simulink library "inp"  (R2021b)
settings: Solver=VariableStepAuto  StartTime=0.0  StopTime=10.0  RelTol=1e-3
undefined symbols (not defined in the file): C_TASK_5MS_S, FALSE, KINP_AcoreReadyToSlp_flg_ovrdflg, KINP_AcoreReadyToSlp_flg_ovrdval, KINP_AllowMovThd_OTA_enum_ovrdflg, KINP_AllowMovThd_OTA_enum_ovrdval, KINP_APSAngleTarget_Deg_ovrdflg, KINP_APSAngleTarget_Deg_ovrdval, KINP_APSDecReq_mps2_ovrdflg, KINP_APSDecReq_mps2_ovrdval, KINP_APSDecReqA_flg_ovrdflg, KINP_APSDecReqA_flg_ovrdval, KINP_APSDFLL_cm_ovrdflg, KINP_APSDFLL_cm_ovrdval, KINP_APSDFLR_cm_ovrdflg, KINP_APSDFLR_cm_ovrdval, KINP_APSDRLL_cm_ovrdflg, KINP_APSDRLL_cm_ovrdval, KINP_APSDRLR_cm_ovrdflg, KINP_APSDRLR_cm_ovrdval, KINP_APSExitCondition_enum_ovrdflg, KINP_APSExitCondition_enum_ovrdval, KINP_APSHWVer_enum_ovrdflg, KINP_APSHWVer_enum_ovrdval, KINP_APSProgressPCT_pct_ovrdflg, KINP_APSProgressPCT_pct_ovrdval, KINP_APSPwrReq_enum_ovrdflg, KINP_APSPwrReq_enum_ovrdval, KINP_APSReq_enum_ovrdflg, KINP_APSReq_enum_ovrdval, KINP_APSRQDisplay_enum_ovrdflg, KINP_APSRQDisplay_enum_ovrdval, KINP_APSRqEPASCtrl_flg_ovrdflg, KINP_APSRqEPASCtrl_flg_ovrdval, KINP_APSShiftPosnReq_enum_ovrdval, KINP_APSShiftPosnReq_enum_ovrflg, KINP_APSSpeedCMD_kph_ovrdval, KINP_APSSpeedCMD_kph_ovrflg, KINP_APSStaSystem_enum_ovrdflg, KINP_APSStaSystem_enum_ovrdval, KINP_APSSWVer_enum_ovrdflg, KINP_APSSWVer_enum_ovrdval, KINP_APSVMCReqA_flg_ovrdval, KINP_APSVMCReqA_flg_ovrflg, KINP_APSVRqEPASCtrl_flg_ovrdflg, KINP_APSVRqEPASCtrl_flg_ovrdval, KINP_AuxBattVolmV_mV_ovrdflg, KINP_AuxBattVolmV_mV_ovrdval, KINP_BTConnectSta_enum_ovrdflg, KINP_BTConnectSta_enum_ovrdval, KINP_CAASSta_enum_ovrdflg, KINP_CAASSta_enum_ovrdval, KINP_CAASVMCReqA_flg_ovrdval, KINP_CAASVMCReqA_flg_ovrflg, KINP_CAN1BusOff_flg_ovrdflg, KINP_CAN1BusOff_flg_ovrdval, KINP_CAN2BusOff_flg_ovrdflg, KINP_CAN2BusOff_flg_ovrdval, KINP_CAN3BusOff_flg_ovrdflg, KINP_CAN3BusOff_flg_ovrdval ... (+222)
libraries: FVT_lib x1035, hcu_lib x1
(part 9 of 33)

== system inp/INP/CAN4/CreateBus ==
  inp_CanValid_bus : Inport
  inp_Hal_bus : Inport  Port=2
  UnitConverter_{1..21,28..30,35,38,45..46,63,65,70..71,74,79..81,83,85..86,88..91,114..116,118..119,121..138,140..142,157,189,192,196..198,201..202,205..206,209..210,213..214,216..250,259..261,267} (122 alike) : DataTypeConversion  OutDataTypeStr=boolean
  UnitConverter_{22..25,31..34,36..37,41..42,47..62,64,69,72..73,76..78,87,94,96,98,100,102,104,106,108,110,112..113,139,147,149,151..156,159,161,163,165,167,169,171,173..177,179,190..191,193..195,200,204,208,212,215,251..258,263,265..266,269,271..272} (93 alike) : DataTypeConversion  OutDataTypeStr=uint8
  UnitConverter_{26..27,40,43..44,75,82,84,93,95,97,99,101,103,105,107,109,111,117,120,143..146,148,150,158,160,162,164,166,168,170,172,178,180..188,199,203,207,211} (48 alike) : DataTypeConversion  OutDataTypeStr=single
  UnitConverter_{39,92,262,264,268,270} (6 alike) : DataTypeConversion  OutDataTypeStr=uint16
  UnitConverter_66 : DataTypeConversion  OutDataTypeStr=uint64
  UnitConverter_67 : DataTypeConversion  OutDataTypeStr=uint64
  UnitConverter_68 : DataTypeConversion  OutDataTypeStr=uint64
  bus_creator : BusCreator  Inputs=272  OutDataTypeStr=Bus: BINP_CAN4_outputs  NonVirtualBus=on
  bus_selector : BusSelector  OutputSignals=VINP_CANMsgValidBodyZoneDR1_flg,VINP_CANMsgValidBodyZoneDR2_flg,VINP_CANMsgValidBodyZonePS1_flg,VINP_CANMsgValidBodyZonePS2_flg,VINP_CANMsgValidDKC1_flg,VINP_CANMsgValidDKC2_flg,VINP_CANMsgValidPTG1_flg,VINP_CANMsgValidZONEDR1_flg,VINP_CANMsgValidZONEDRVCU_flg,VINP_CANMsgValidZONEFR1_flg,VINP_CANMsgValidZONEFRVCU_flg,VINP_CANMsgValidzGWAPTC1_flg,VINP_CANMsgValidzGWCANFr1_flg,VINP_CANMsgValidzGWLINDr1_flg,VINP_CANMsgValidzGWLINDr2_flg,VINP_CANMsgValidzGWLINFr1_flg,VINP_CANMsgValidzGWLINFr2_flg,VINP_CANMsgValidzGWSEAT1_flg
  bus_selector_1 : BusSelector  OutputSignals=VINP_BDDSEATAntiSta_flg,VINP_BDDSEATEntryFunSta_flg,VINP_BDDSEATErrorSta_flg,VINP_BDDSEATMemSetSta_enum,VINP_BDDSEATModeSta_enum,VINP_BDDSEATVentSta_enum,VINP_BDDSEATheaterSta_enum,VINP_BDAPMWinFOpenedSta_pct,VINP_BDAPMWinROpenedSta_pct,VINP_BDDoorFHandleCloseSta_flg,VINP_BDDoorRHandleCloseSta_flg,VINP_BPPSEATErrorSta_flg,VINP_BPPSEATModeSta_enum,VINP_BPPSEATVentSta_enum,VINP_BPPSEATheaterSta_enum,VINP_BPPTGActiveSta_enum,VINP_BPPTGExistSta_flg,VINP_BPPTGInsideSW1Sta_enum,VINP_BPPTGInsideSW2Sta_enum,VINP_BPPTGIsSetHeightSta_flg,VINP_BPPTGLeftHallPosnSta_enum,VINP_BPPTGOpenRatioSta_pct,VINP_BPPTGRDILCmd_enum,VINP_BPPTGSysSta_enum,VINP_BPAPMWinFOpenedSta_pct,VINP_BPAPMWinROpenedSta_pct,VINP_BPDoorFHandleCloseSta_flg,VINP_BPDoorRHandleCloseSta_flg,VINP_BPSEATLVentSta_enum,VINP_BPSEATMLVentSta_enum,VINP_BPSEATMRVentSta_enum,VINP_BPSEATRVentSta_enum,VINP_DKCKeyNumSta_enum,VINP_DKCKeyTypeSta_enum,VINP_DKCPDkeyAreaRAPSSta_enum,VINP_DKCParkingModeCmd_enum,VINP_DKCReVehData_enum,VINP_PCommandToBCM_enum,VINP_PCommandToPTG_enum,VINP_PDKeyAreaLockUnlock_enum,VINP_PDKeyAreaPS_enum,VINP_PDKeyAreaPTG_enum,VINP_PDKeyWelcome_enum,VINP_PDkeyShowIVI_enum,VINP_PKeyMiss_flg,VINP_PKeyMode_enum,VINP_PUIDLowPower_flg,VINP_EncryptionDATA063_enum,VINP_EncryptionDATA64127_enum,VINP_RandomNumberX_enum,VINP_PTGActiveSta_enum,VINP_PTGAutoStaus_flg,VINP_PTGExist_flg,VINP_PTGHWVer_enum,VINP_PTGInnerSW2_enum,VINP_PTGIsSetHeight_flg,VINP_PTGOpenRatio_pct,VINP_PTGRDILSta_enum,VINP_PTGSWVer_enum,VINP_PTGSysSta_enum,VINP_DrLockSta_flg,VINP_MIRRORFOLDSW_flg,VINP_RLTurnLPErr_flg,VINP_RLTurnLampC_mA,VINP_RRTurnLPErr_flg,VINP_RRTurnLampC_mA,VINP_RWiperAS_flg,VINP_RWiperProtection_flg,VINP_BlowerErr_enum,VINP_DrPMMLVOutPErrLmp_flg,VINP_DrPMMSysErrLmp_flg,VINP_DrSCPSysErrLmp_flg,VINP_DrStdAErrSta_flg,VINP_LeftHallPos_enum,VINP_SolarL_W,VINP_SolarLErr_enum,VINP_SolarR_W,VINP_SolarRErr_enum,VINP_TFaceL_C,VINP_TFaceLErr_enum,VINP_TFaceR_C,VINP_TFaceRErr_enum,VINP_TFaceRr_C,VINP_TFaceRrErr_enum,VINP_TFootL_C,VINP_TFootLErr_enum,VINP_TFootR_C,VINP_TFootRErr_enum,VINP_TFootRr_C,VINP_TFootRrErr_enum,VINP_Tevap_C,VINP_TevapErr_enum,VINP_Tincar_C,VINP_TincarErr_enum,VINP_ZoneDrMalfunLevel_enum,VINP_ChargeInletLockSta_flg,VINP_CompProEN_flg,VINP_FLTurnLPErr_flg,VINP_FLTurnLampC_mA,VINP_FLTurnLightWarning_flg,VINP_FRTurnLPErr_flg,VINP_FRTurnLampC_mA,VINP_FRTurnLightWarning_flg,VINP_FWiperAS_flg,VINP_FWiperProtection_flg,VINP_LADBHibeamIndication_flg,VINP_LADBOperationStatus_flg,VINP_LADBWarning_flg,VINP_LAHBWarning_flg,VINP_LDRLWarning_flg,VINP_LLBWarning_flg,VINP_LpositionLampWarning_flg,VINP_RADBHibeamIndication_flg,VINP_RADBOperationStatus_flg,VINP_RADBWarning_flg,VINP_RAHBWarning_flg,VINP_RDRLWarning_flg,VINP_RLBWarning_flg,VINP_RpositionLampWarning_flg,VINP_TrailerCheck_flg,VINP_TrailerModeSta_enum,VINP_ZFRBCMChargerDoorSWSta_flg,VINP_ZFRBCMHRLTurnLPNormalSta_flg,VINP_ZFRBCMHRRTurnLPHNormalSta_flg,VINP_ZFRTHCMCLEVentActYSta_pct,VINP_ZFRTHCMCREVentActYSta_pct,VINP_ZFRTHCMLEVentActYSta_pct,VINP_ZFRTHCMREVentActYSta_pct,VINP_AGSErr_enum,VINP_BatInTemp_C,VINP_BatInTempErr_enum,VINP_BatOutTemp_C,VINP_COMPErr_enum,VINP_EACProtectEnable_enum,VINP_EWP3Err_enum,VINP_EXV1Err_enum,VINP_EXV2Err_enum,VINP_FanErr_enum,VINP_FrPMMLimpHomeActReq_flg,VINP_MotorInTemp_C,VINP_MotorInTempErr_enum,VINP_MotorOutTemp_C,VINP_MotorOutTempErr_enum,VINP_PTHighP_KPa,VINP_PTHighPErr_enum,VINP_PTHighTact_C,VINP_PTHighTactErr_enum,VINP_PTLowP1_KPa,VINP_PTLowP1Err_enum,VINP_PTLowP2_KPa,VINP_PTLowP2Err_enum,VINP_PTLowT1_C,VINP_PTLowT1Err_enum,VINP_PTLowT2_C,VINP_PTLowT2Err_enum,VINP_SOTXVErr_enum,VINP_SOV1Err_enum,VINP_SOV2Err_enum,VINP_SOV3Err_enum,VINP_Tamb_C,VINP_TambErr_enum,VINP_FrntPTCLeActHeatPwr_W,VINP_FrntPTCRearLeActHeatPwr_W,VINP_FrntPTCRearRiActHeatPwr_W,VINP_FrntPTCRiActHeatPwr_W,VINP_COMPActualPwr_W,VINP_COMPConCur_A,VINP_COMPConVolt_V,VINP_COMPStatorSpd_rpm,VINP_PTC1PowerConsumption_kW,VINP_CSWDimSw_flg,VINP_CSWFWasSwSta_enum,VINP_CSWFWipSwSta_enum,VINP_CSWPassSWSta_flg,VINP_CSWRWasSWSta_enum,VINP_CSWRWipIntSwSta_enum,VINP_CSWTurnSwSta_enum,VINP_FAPWL01LINResponseError_flg,VINP_LDrvMotorRelayError_flg,VINP_LDrvMotorRippleError_flg,VINP_LDrvValWdwOpened_pct,VINP_LDrvWdwPositionSts_enum,VINP_LPasMotorRelayError_flg,VINP_LPasMotorRippleError_flg,VINP_LPasValWdwOpened_pct,VINP_LPasWdwPositionSts_enum,VINP_LRLDMotorRelayError_flg,VINP_LRLDMotorRippleError_flg,VINP_LRLDValWdwOpened_pct,VINP_LRLDWdwPositionSts_enum,VINP_LRRDMotorRelayError_flg,VINP_LRRDMotorRippleError_flg,VINP_LRRDValWdwOpened_pct,VINP_LRRDWdwPositionSts_enum,VINP_RAPWL01LINResponseError_flg,VINP_RLSLampSta_flg,VINP_RLSRainSnrWiperCmd_enum,VINP_SWC2LADASSta_flg,VINP_SWC2LDriveModeSta_flg,VINP_SWC2LHomeSta_flg,VINP_SWC2LLeftSta_flg,VINP_SWC2LRegenUpSta_flg,VINP_SWC2LRightSta_flg,VINP_SWC2LScrollDownSta_flg,VINP_SWC2LScrollPressSta_flg,VINP_SWC2LScrollUpSta_flg,VINP_SWC2RCustomizeSta_flg,VINP_SWC2RLeftSta_flg,VINP_SWC2RPageSwitchSta_flg,VINP_SWC2RRegenDownSta_flg,VINP_SWC2RRightSta_flg,VINP_SWC2RScrollDownSta_flg,VINP_SWC2RScrollPressSta_flg,VINP_SWC2RScrollUpSta_flg,VINP_SWC2RVRSta_flg,VINP_SWCACCSta_flg,VINP_SWCCANCELSta_flg,VINP_SWCDistanceSta_flg,VINP_SWCDownSta_flg,VINP_SWCLKASta_flg,VINP_SWCLeftSta_flg,VINP_SWCRegenDown_flg,VINP_SWCRegenUp_flg,VINP_SWCResUpSta_flg,VINP_SWCRightSta_flg,VINP_SWCSetdownSta_flg,VINP_SWCTripSta_flg,VINP_SWCUndefinedSta_flg,VINP_SWCUpSta_flg,VINP_SWCVRSta_flg,VINP_SWCmodeSta_flg,VINP_ACT1ResponseError_flg,VINP_AGSActualPosition_enum,VINP_FGSIntenRspSta_enum,VINP_EWP1BlockError_enum,VINP_EWP1OverCurrError_enum,VINP_EWP2BlockError_enum,VINP_EWP2OverCurrError_enum,VINP_EWP3BlockError_enum,VINP_EWP3OverCurrError_enum,VINP_DSEATAntiSta_flg,VINP_DSEATEntryFunSta_flg,VINP_DSEATErrorSta_flg,VINP_DSEATHWVer_enum,VINP_DSEATMode_enum,VINP_DSEATSWVer_enum,VINP_DSEATVentSta_enum,VINP_DSEATheatersta_enum,VINP_PSEATErrorSta_flg,VINP_PSEATHWVer_enum,VINP_PSEATMode_enum,VINP_PSEATSWVer_enum,VINP_PSEATVentSta_enum,VINP_PSEATheatersta_enum
  BINP_outputs : Outport
  wires:
  inp_CanValid_bus/1 -> [inp_CanValid_bus]
  inp_Hal_bus/1 -> [inp_Hal_bus]
  bus_selector/1 -> UnitConverter_1/1  "<VINP_CANMsgValidBodyZoneDR1_flg>"
  UnitConverter_1/1 -> bus_creator/1  "VINP_CANMsgValidBodyZoneDR1_flg"
  bus_selector/2 -> UnitConverter_2/1  "<VINP_CANMsgValidBodyZoneDR2_flg>"
  UnitConverter_2/1 -> bus_creator/2  "VINP_CANMsgValidBodyZoneDR2_flg"
  bus_selector/3 -> UnitConverter_3/1  "<VINP_CANMsgValidBodyZonePS1_flg>"
  UnitConverter_3/1 -> bus_creator/3  "VINP_CANMsgValidBodyZonePS1_flg"
  bus_selector/4 -> UnitConverter_4/1  "<VINP_CANMsgValidBodyZonePS2_flg>"
  UnitConverter_4/1 -> bus_creator/4  "VINP_CANMsgValidBodyZonePS2_flg"
  bus_selector/5 -> UnitConverter_5/1  "<VINP_CANMsgValidDKC1_flg>"
  UnitConverter_5/1 -> bus_creator/5  "VINP_CANMsgValidDKC1_flg"
  bus_selector/6 -> UnitConverter_6/1  "<VINP_CANMsgValidDKC2_flg>"
  UnitConverter_6/1 -> bus_creator/6  "VINP_CANMsgValidDKC2_flg"
  bus_selector/7 -> UnitConverter_7/1  "<VINP_CANMsgValidPTG1_flg>"
  UnitConverter_7/1 -> bus_creator/7  "VINP_CANMsgValidPTG1_flg"
  bus_selector/8 -> UnitConverter_8/1  "<VINP_CANMsgValidZONEDR1_flg>"
  UnitConverter_8/1 -> bus_creator/8  "VINP_CANMsgValidZONEDR1_flg"
  bus_selector/9 -> UnitConverter_9/1  "<VINP_CANMsgValidZONEDRVCU_flg>"
  UnitConverter_9/1 -> bus_creator/9  "VINP_CANMsgValidZONEDRVCU_flg"
  bus_selector/10 -> UnitConverter_10/1  "<VINP_CANMsgValidZONEFR1_flg>"
  UnitConverter_10/1 -> bus_creator/10  "VINP_CANMsgValidZONEFR1_flg"
  bus_selector/11 -> UnitConverter_11/1  "<VINP_CANMsgValidZONEFRVCU_flg>"
  UnitConverter_11/1 -> bus_creator/11  "VINP_CANMsgValidZONEFRVCU_flg"
  bus_selector/12 -> UnitConverter_12/1  "<VINP_CANMsgValidzGWAPTC1_flg>"
  UnitConverter_12/1 -> bus_creator/12  "VINP_CANMsgValidzGWAPTC1_flg"
  bus_selector/13 -> UnitConverter_13/1  "<VINP_CANMsgValidzGWCANFr1_flg>"
  UnitConverter_13/1 -> bus_creator/13  "VINP_CANMsgValidzGWCANFr1_flg"
  bus_selector/14 -> UnitConverter_14/1  "<VINP_CANMsgValidzGWLINDr1_flg>"
  UnitConverter_14/1 -> bus_creator/14  "VINP_CANMsgValidzGWLINDr1_flg"
  bus_selector/15 -> UnitConverter_15/1  "<VINP_CANMsgValidzGWLINDr2_flg>"
  UnitConverter_15/1 -> bus_creator/15  "VINP_CANMsgValidzGWLINDr2_flg"
  bus_selector/16 -> UnitConverter_16/1  "<VINP_CANMsgValidzGWLINFr1_flg>"
  UnitConverter_16/1 -> bus_creator/16  "VINP_CANMsgValidzGWLINFr1_flg"
  bus_selector/17 -> UnitConverter_17/1  "<VINP_CANMsgValidzGWLINFr2_flg>"
  UnitConverter_17/1 -> bus_creator/17  "VINP_CANMsgValidzGWLINFr2_flg"
  bus_selector/18 -> UnitConverter_18/1  "<VINP_CANMsgValidzGWSEAT1_flg>"
  UnitConverter_18/1 -> bus_creator/18  "VINP_CANMsgValidzGWSEAT1_flg"
  bus_selector_1/1 -> UnitConverter_19/1  "<VINP_BDDSEATAntiSta_flg>"
  UnitConverter_19/1 -> bus_creator/19  "VINP_BDDSEATAntiSta_flg"
  bus_selector_1/2 -> UnitConverter_20/1  "<VINP_BDDSEATEntryFunSta_flg>"
  UnitConverter_20/1 -> bus_creator/20  "VINP_BDDSEATEntryFunSta_flg"
  bus_selector_1/3 -> UnitConverter_21/1  "<VINP_BDDSEATErrorSta_flg>"
  UnitConverter_21/1 -> bus_creator/21  "VINP_BDDSEATErrorSta_flg"
  bus_selector_1/4 -> UnitConverter_22/1  "<VINP_BDDSEATMemSetSta_enum>"
  UnitConverter_22/1 -> bus_creator/22  "VINP_BDDSEATMemSetSta_enum"
  bus_selector_1/5 -> UnitConverter_23/1  "<VINP_BDDSEATModeSta_enum>"
  UnitConverter_23/1 -> bus_creator/23  "VINP_BDDSEATModeSta_enum"
  bus_selector_1/6 -> UnitConverter_24/1  "<VINP_BDDSEATVentSta_enum>"
  UnitConverter_24/1 -> bus_creator/24  "VINP_BDDSEATVentSta_enum"
  bus_selector_1/7 -> UnitConverter_25/1  "<VINP_BDDSEATheaterSta_enum>"
  UnitConverter_25/1 -> bus_creator/25  "VINP_BDDSEATheaterSta_enum"
  bus_selector_1/8 -> UnitConverter_26/1  "<VINP_BDAPMWinFOpenedSta_pct>"
  UnitConverter_26/1 -> bus_creator/26  "VINP_BDAPMWinFOpenedSta_pct"
  bus_selector_1/9 -> UnitConverter_27/1  "<VINP_BDAPMWinROpenedSta_pct>"
  UnitConverter_27/1 -> bus_creator/27  "VINP_BDAPMWinROpenedSta_pct"
  bus_selector_1/10 -> UnitConverter_28/1  "<VINP_BDDoorFHandleCloseSta_flg>"
  UnitConverter_28/1 -> bus_creator/28  "VINP_BDDoorFHandleCloseSta_flg"
  bus_selector_1/11 -> UnitConverter_29/1  "<VINP_BDDoorRHandleCloseSta_flg>"
  UnitConverter_29/1 -> bus_creator/29  "VINP_BDDoorRHandleCloseSta_flg"
  bus_selector_1/12 -> UnitConverter_30/1  "<VINP_BPPSEATErrorSta_flg>"
  UnitConverter_30/1 -> bus_creator/30  "VINP_BPPSEATErrorSta_flg"
  bus_selector_1/13 -> UnitConverter_31/1  "<VINP_BPPSEATModeSta_enum>"
  UnitConverter_31/1 -> bus_creator/31  "VINP_BPPSEATModeSta_enum"
  bus_selector_1/14 -> UnitConverter_32/1  "<VINP_BPPSEATVentSta_enum>"
  UnitConverter_32/1 -> bus_creator/32  "VINP_BPPSEATVentSta_enum"
  bus_selector_1/15 -> UnitConverter_33/1  "<VINP_BPPSEATheaterSta_enum>"
  UnitConverter_33/1 -> bus_creator/33  "VINP_BPPSEATheaterSta_enum"
  bus_selector_1/16 -> UnitConverter_34/1  "<VINP_BPPTGActiveSta_enum>"
  UnitConverter_34/1 -> bus_creator/34  "VINP_BPPTGActiveSta_enum"
  bus_selector_1/17 -> UnitConverter_35/1  "<VINP_BPPTGExistSta_flg>"
  UnitConverter_35/1 -> bus_creator/35  "VINP_BPPTGExistSta_flg"
  bus_selector_1/18 -> UnitConverter_36/1  "<VINP_BPPTGInsideSW1Sta_enum>"
  UnitConverter_36/1 -> bus_creator/36  "VINP_BPPTGInsideSW1Sta_enum"
  bus_selector_1/19 -> UnitConverter_37/1  "<VINP_BPPTGInsideSW2Sta_enum>"
  UnitConverter_37/1 -> bus_creator/37  "VINP_BPPTGInsideSW2Sta_enum"
  bus_selector_1/20 -> UnitConverter_38/1  "<VINP_BPPTGIsSetHeightSta_flg>"
  UnitConverter_38/1 -> bus_creator/38  "VINP_BPPTGIsSetHeightSta_flg"
  bus_selector_1/21 -> UnitConverter_39/1  "<VINP_BPPTGLeftHallPosnSta_enum>"
  UnitConverter_39/1 -> bus_creator/39  "VINP_BPPTGLeftHallPosnSta_enum"
  bus_selector_1/22 -> UnitConverter_40/1  "<VINP_BPPTGOpenRatioSta_pct>"
  UnitConverter_40/1 -> bus_creator/40  "VINP_BPPTGOpenRatioSta_pct"
  bus_selector_1/23 -> UnitConverter_41/1  "<VINP_BPPTGRDILCmd_enum>"
  UnitConverter_41/1 -> bus_creator/41  "VINP_BPPTGRDILCmd_enum"
  bus_selector_1/24 -> UnitConverter_42/1  "<VINP_BPPTGSysSta_enum>"
  UnitConverter_42/1 -> bus_creator/42  "VINP_BPPTGSysSta_enum"
  bus_selector_1/25 -> UnitConverter_43/1  "<VINP_BPAPMWinFOpenedSta_pct>"
  UnitConverter_43/1 -> bus_creator/43  "VINP_BPAPMWinFOpenedSta_pct"
  bus_selector_1/26 -> UnitConverter_44/1  "<VINP_BPAPMWinROpenedSta_pct>"
  UnitConverter_44/1 -> bus_creator/44  "VINP_BPAPMWinROpenedSta_pct"
  bus_selector_1/27 -> UnitConverter_45/1  "<VINP_BPDoorFHandleCloseSta_flg>"
  UnitConverter_45/1 -> bus_creator/45  "VINP_BPDoorFHandleCloseSta_flg"
  bus_selector_1/28 -> UnitConverter_46/1  "<VINP_BPDoorRHandleCloseSta_flg>"
  UnitConverter_46/1 -> bus_creator/46  "VINP_BPDoorRHandleCloseSta_flg"
  bus_selector_1/29 -> UnitConverter_47/1  "<VINP_BPSEATLVentSta_enum>"
  UnitConverter_47/1 -> bus_creator/47  "VINP_BPSEATLVentSta_enum"
  bus_selector_1/30 -> UnitConverter_48/1  "<VINP_BPSEATMLVentSta_enum>"
  UnitConverter_48/1 -> bus_creator/48  "VINP_BPSEATMLVentSta_enum"
  bus_selector_1/31 -> UnitConverter_49/1  "<VINP_BPSEATMRVentSta_enum>"
  UnitConverter_49/1 -> bus_creator/49  "VINP_BPSEATMRVentSta_enum"
  bus_selector_1/32 -> UnitConverter_50/1  "<VINP_BPSEATRVentSta_enum>"
  UnitConverter_50/1 -> bus_creator/50  "VINP_BPSEATRVentSta_enum"
  bus_selector_1/33 -> UnitConverter_51/1  "<VINP_DKCKeyNumSta_enum>"
  UnitConverter_51/1 -> bus_creator/51  "VINP_DKCKeyNumSta_enum"
  bus_selector_1/34 -> UnitConverter_52/1  "<VINP_DKCKeyTypeSta_enum>"
  UnitConverter_52/1 -> bus_creator/52  "VINP_DKCKeyTypeSta_enum"
  bus_selector_1/35 -> UnitConverter_53/1  "<VINP_DKCPDkeyAreaRAPSSta_enum>"
  UnitConverter_53/1 -> bus_creator/53  "VINP_DKCPDkeyAreaRAPSSta_enum"
  bus_selector_1/36 -> UnitConverter_54/1  "<VINP_DKCParkingModeCmd_enum>"
  UnitConverter_54/1 -> bus_creator/54  "VINP_DKCParkingModeCmd_enum"
  bus_selector_1/37 -> UnitConverter_55/1  "<VINP_DKCReVehData_enum>"
  UnitConverter_55/1 -> bus_creator/55  "VINP_DKCReVehData_enum"
  bus_selector_1/38 -> UnitConverter_56/1  "<VINP_PCommandToBCM_enum>"
  UnitConverter_56/1 -> bus_creator/56  "VINP_PCommandToBCM_enum"
  bus_selector_1/39 -> UnitConverter_57/1  "<VINP_PCommandToPTG_enum>"
  UnitConverter_57/1 -> bus_creator/57  "VINP_PCommandToPTG_enum"
  bus_selector_1/40 -> UnitConverter_58/1  "<VINP_PDKeyAreaLockUnlock_enum>"
  UnitConverter_58/1 -> bus_creator/58  "VINP_PDKeyAreaLockUnlock_enum"
  bus_selector_1/41 -> UnitConverter_59/1  "<VINP_PDKeyAreaPS_enum>"
  UnitConverter_59/1 -> bus_creator/59  "VINP_PDKeyAreaPS_enum"
  bus_selector_1/42 -> UnitConverter_60/1  "<VINP_PDKeyAreaPTG_enum>"
  UnitConverter_60/1 -> bus_creator/60  "VINP_PDKeyAreaPTG_enum"
  bus_selector_1/43 -> UnitConverter_61/1  "<VINP_PDKeyWelcome_enum>"
  UnitConverter_61/1 -> bus_creator/61  "VINP_PDKeyWelcome_enum"
  bus_selector_1/44 -> UnitConverter_62/1  "<VINP_PDkeyShowIVI_enum>"
  UnitConverter_62/1 -> bus_creator/62  "VINP_PDkeyShowIVI_enum"
  bus_selector_1/45 -> UnitConverter_63/1  "<VINP_PKeyMiss_flg>"
  UnitConverter_63/1 -> bus_creator/63  "VINP_PKeyMiss_flg"
  bus_selector_1/46 -> UnitConverter_64/1  "<VINP_PKeyMode_enum>"
  UnitConverter_64/1 -> bus_creator/64  "VINP_PKeyMode_enum"
  bus_selector_1/47 -> UnitConverter_65/1  "<VINP_PUIDLowPower_flg>"
  UnitConverter_65/1 -> bus_creator/65  "VINP_PUIDLowPower_flg"
  bus_selector_1/48 -> UnitConverter_66/1  "<VINP_EncryptionDATA063_enum>"
  UnitConverter_66/1 -> bus_creator/66  "VINP_EncryptionDATA063_enum"
  bus_selector_1/49 -> UnitConverter_67/1  "<VINP_EncryptionDATA64127_enum>"
  UnitConverter_67/1 -> bus_creator/67  "VINP_EncryptionDATA64127_enum"
  bus_selector_1/50 -> UnitConverter_68/1  "<VINP_RandomNumberX_enum>"
  UnitConverter_68/1 -> bus_creator/68  "VINP_RandomNumberX_enum"
  bus_selector_1/51 -> UnitConverter_69/1  "<VINP_PTGActiveSta_enum>"
  UnitConverter_69/1 -> bus_creator/69  "VINP_PTGActiveSta_enum"
  bus_selector_1/52 -> UnitConverter_70/1  "<VINP_PTGAutoStaus_flg>"
  UnitConverter_70/1 -> bus_creator/70  "VINP_PTGAutoStaus_flg"
  bus_selector_1/53 -> UnitConverter_71/1  "<VINP_PTGExist_flg>"
  UnitConverter_71/1 -> bus_creator/71  "VINP_PTGExist_flg"
  bus_selector_1/54 -> UnitConverter_72/1  "<VINP_PTGHWVer_enum>"
  UnitConverter_72/1 -> bus_creator/72  "VINP_PTGHWVer_enum"
  bus_selector_1/55 -> UnitConverter_73/1  "<VINP_PTGInnerSW2_enum>"
  UnitConverter_73/1 -> bus_creator/73  "VINP_PTGInnerSW2_enum"
  bus_selector_1/56 -> UnitConverter_74/1  "<VINP_PTGIsSetHeight_flg>"
  UnitConverter_74/1 -> bus_creator/74  "VINP_PTGIsSetHeight_flg"
  bus_selector_1/57 -> UnitConverter_75/1  "<VINP_PTGOpenRatio_pct>"
  UnitConverter_75/1 -> bus_creator/75  "VINP_PTGOpenRatio_pct"
  bus_selector_1/58 -> UnitConverter_76/1  "<VINP_PTGRDILSta_enum>"
  UnitConverter_76/1 -> bus_creator/76  "VINP_PTGRDILSta_enum"
  bus_selector_1/59 -> UnitConverter_77/1  "<VINP_PTGSWVer_enum>"
  UnitConverter_77/1 -> bus_creator/77  "VINP_PTGSWVer_enum"
  bus_selector_1/60 -> UnitConverter_78/1  "<VINP_PTGSysSta_enum>"
  UnitConverter_78/1 -> bus_creator/78  "VINP_PTGSysSta_enum"
  bus_selector_1/61 -> UnitConverter_79/1  "<VINP_DrLockSta_flg>"
  UnitConverter_79/1 -> bus_creator/79  "VINP_DrLockSta_flg"
  bus_selector_1/62 -> UnitConverter_80/1  "<VINP_MIRRORFOLDSW_flg>"
  UnitConverter_80/1 -> bus_creator/80  "VINP_MIRRORFOLDSW_flg"
  bus_selector_1/63 -> UnitConverter_81/1  "<VINP_RLTurnLPErr_flg>"
  UnitConverter_81/1 -> bus_creator/81  "VINP_RLTurnLPErr_flg"
  bus_selector_1/64 -> UnitConverter_82/1  "<VINP_RLTurnLampC_mA>"
  UnitConverter_82/1 -> bus_creator/82  "VINP_RLTurnLampC_mA"
  bus_selector_1/65 -> UnitConverter_83/1  "<VINP_RRTurnLPErr_flg>"
  UnitConverter_83/1 -> bus_creator/83  "VINP_RRTurnLPErr_flg"
  bus_selector_1/66 -> UnitConverter_84/1  "<VINP_RRTurnLampC_mA>"
  UnitConverter_84/1 -> bus_creator/84  "VINP_RRTurnLampC_mA"
  bus_selector_1/67 -> UnitConverter_85/1  "<VINP_RWiperAS_flg>"
  UnitConverter_85/1 -> bus_creator/85  "VINP_RWiperAS_flg"
  bus_selector_1/68 -> UnitConverter_86/1  "<VINP_RWiperProtection_flg>"
  UnitConverter_86/1 -> bus_creator/86  "VINP_RWiperProtection_flg"
  bus_selector_1/69 -> UnitConverter_87/1  "<VINP_BlowerErr_enum>"
  UnitConverter_87/1 -> bus_creator/87  "VINP_BlowerErr_enum"
  bus_selector_1/70 -> UnitConverter_88/1  "<VINP_DrPMMLVOutPErrLmp_flg>"
  UnitConverter_88/1 -> bus_creator/88  "VINP_DrPMMLVOutPErrLmp_flg"
  bus_selector_1/71 -> UnitConverter_89/1  "<VINP_DrPMMSysErrLmp_flg>"
  UnitConverter_89/1 -> bus_creator/89  "VINP_DrPMMSysErrLmp_flg"
  bus_selector_1/72 -> UnitConverter_90/1  "<VINP_DrSCPSysErrLmp_flg>"
  UnitConverter_90/1 -> bus_creator/90  "VINP_DrSCPSysErrLmp_flg"
  bus_selector_1/73 -> UnitConverter_91/1  "<VINP_DrStdAErrSta_flg>"
  UnitConverter_91/1 -> bus_creator/91  "VINP_DrStdAErrSta_flg"
  bus_selector_1/74 -> UnitConverter_92/1  "<VINP_LeftHallPos_enum>"
  UnitConverter_92/1 -> bus_creator/92  "VINP_LeftHallPos_enum"
  bus_selector_1/75 -> UnitConverter_93/1  "<VINP_SolarL_W>"
  UnitConverter_93/1 -> bus_creator/93  "VINP_SolarL_W"
  bus_selector_1/76 -> UnitConverter_94/1  "<VINP_SolarLErr_enum>"
  UnitConverter_94/1 -> bus_creator/94  "VINP_SolarLErr_enum"
  bus_selector_1/77 -> UnitConverter_95/1  "<VINP_SolarR_W>"
  UnitConverter_95/1 -> bus_creator/95  "VINP_SolarR_W"
  bus_selector_1/78 -> UnitConverter_96/1  "<VINP_SolarRErr_enum>"
  UnitConverter_96/1 -> bus_creator/96  "VINP_SolarRErr_enum"
  bus_selector_1/79 -> UnitConverter_97/1  "<VINP_TFaceL_C>"
  UnitConverter_97/1 -> bus_creator/97  "VINP_TFaceL_C"
  bus_selector_1/80 -> UnitConverter_98/1  "<VINP_TFaceLErr_enum>"
  UnitConverter_98/1 -> bus_creator/98  "VINP_TFaceLErr_enum"
  bus_selector_1/81 -> UnitConverter_99/1  "<VINP_TFaceR_C>"
  UnitConverter_99/1 -> bus_creator/99  "VINP_TFaceR_C"
  bus_selector_1/82 -> UnitConverter_100/1  "<VINP_TFaceRErr_enum>"
  UnitConverter_100/1 -> bus_creator/100  "VINP_TFaceRErr_enum"
  bus_selector_1/83 -> UnitConverter_101/1  "<VINP_TFaceRr_C>"
  UnitConverter_101/1 -> bus_creator/101  "VINP_TFaceRr_C"
  bus_selector_1/84 -> UnitConverter_102/1  "<VINP_TFaceRrErr_enum>"
  UnitConverter_102/1 -> bus_creator/102  "VINP_TFaceRrErr_enum"
  bus_selector_1/85 -> UnitConverter_103/1  "<VINP_TFootL_C>"
  UnitConverter_103/1 -> bus_creator/103  "VINP_TFootL_C"
  bus_selector_1/86 -> UnitConverter_104/1  "<VINP_TFootLErr_enum>"
  UnitConverter_104/1 -> bus_creator/104  "VINP_TFootLErr_enum"
  bus_selector_1/87 -> UnitConverter_105/1  "<VINP_TFootR_C>"
  UnitConverter_105/1 -> bus_creator/105  "VINP_TFootR_C"
  bus_selector_1/88 -> UnitConverter_106/1  "<VINP_TFootRErr_enum>"
  UnitConverter_106/1 -> bus_creator/106  "VINP_TFootRErr_enum"
  bus_selector_1/89 -> UnitConverter_107/1  "<VINP_TFootRr_C>"
  UnitConverter_107/1 -> bus_creator/107  "VINP_TFootRr_C"
  bus_selector_1/90 -> UnitConverter_108/1  "<VINP_TFootRrErr_enum>"
  UnitConverter_108/1 -> bus_creator/108  "VINP_TFootRrErr_enum"
  bus_selector_1/91 -> UnitConverter_109/1  "<VINP_Tevap_C>"
  UnitConverter_109/1 -> bus_creator/109  "VINP_Tevap_C"
  bus_selector_1/92 -> UnitConverter_110/1  "<VINP_TevapErr_enum>"
  UnitConverter_110/1 -> bus_creator/110  "VINP_TevapErr_enum"
  bus_selector_1/93 -> UnitConverter_111/1  "<VINP_Tincar_C>"
  UnitConverter_111/1 -> bus_creator/111  "VINP_Tincar_C"
  bus_selector_1/94 -> UnitConverter_112/1  "<VINP_TincarErr_enum>"
  UnitConverter_112/1 -> bus_creator/112  "VINP_TincarErr_enum"
  bus_selector_1/95 -> UnitConverter_113/1  "<VINP_ZoneDrMalfunLevel_enum>"
  UnitConverter_113/1 -> bus_creator/113  "VINP_ZoneDrMalfunLevel_enum"
  bus_selector_1/96 -> UnitConverter_114/1  "<VINP_ChargeInletLockSta_flg>"
  UnitConverter_114/1 -> bus_creator/114  "VINP_ChargeInletLockSta_flg"
  bus_selector_1/97 -> UnitConverter_115/1  "<VINP_CompProEN_flg>"
  UnitConverter_115/1 -> bus_creator/115  "VINP_CompProEN_flg"
  bus_selector_1/98 -> UnitConverter_116/1  "<VINP_FLTurnLPErr_flg>"
  UnitConverter_116/1 -> bus_creator/116  "VINP_FLTurnLPErr_flg"
  bus_selector_1/99 -> UnitConverter_117/1  "<VINP_FLTurnLampC_mA>"
  UnitConverter_117/1 -> bus_creator/117  "VINP_FLTurnLampC_mA"
  bus_selector_1/100 -> UnitConverter_118/1  "<VINP_FLTurnLightWarning_flg>"
  UnitConverter_118/1 -> bus_creator/118  "VINP_FLTurnLightWarning_flg"
  bus_selector_1/101 -> UnitConverter_119/1  "<VINP_FRTurnLPErr_flg>"
  UnitConverter_119/1 -> bus_creator/119  "VINP_FRTurnLPErr_flg"
  bus_selector_1/102 -> UnitConverter_120/1  "<VINP_FRTurnLampC_mA>"
  UnitConverter_120/1 -> bus_creator/120  "VINP_FRTurnLampC_mA"
  bus_selector_1/103 -> UnitConverter_121/1  "<VINP_FRTurnLightWarning_flg>"
  UnitConverter_121/1 -> bus_creator/121  "VINP_FRTurnLightWarning_flg"
  bus_selector_1/104 -> UnitConverter_122/1  "<VINP_FWiperAS_flg>"
  UnitConverter_122/1 -> bus_creator/122  "VINP_FWiperAS_flg"
  bus_selector_1/105 -> UnitConverter_123/1  "<VINP_FWiperProtection_flg>"
  UnitConverter_123/1 -> bus_creator/123  "VINP_FWiperProtection_flg"
  bus_selector_1/106 -> UnitConverter_124/1  "<VINP_LADBHibeamIndication_flg>"
  UnitConverter_124/1 -> bus_creator/124  "VINP_LADBHibeamIndication_flg"
  bus_selector_1/107 -> UnitConverter_125/1  "<VINP_LADBOperationStatus_flg>"
  UnitConverter_125/1 -> bus_creator/125  "VINP_LADBOperationStatus_flg"
  bus_selector_1/108 -> UnitConverter_126/1  "<VINP_LADBWarning_flg>"
  UnitConverter_126/1 -> bus_creator/126  "VINP_LADBWarning_flg"
  bus_selector_1/109 -> UnitConverter_127/1  "<VINP_LAHBWarning_flg>"
  UnitConverter_127/1 -> bus_creator/127  "VINP_LAHBWarning_flg"
  bus_selector_1/110 -> UnitConverter_128/1  "<VINP_LDRLWarning_flg>"
  UnitConverter_128/1 -> bus_creator/128  "VINP_LDRLWarning_flg"
  bus_selector_1/111 -> UnitConverter_129/1  "<VINP_LLBWarning_flg>"
  UnitConverter_129/1 -> bus_creator/129  "VINP_LLBWarning_flg"
  bus_selector_1/112 -> UnitConverter_130/1  "<VINP_LpositionLampWarning_flg>"
  UnitConverter_130/1 -> bus_creator/130  "VINP_LpositionLampWarning_flg"
  bus_selector_1/113 -> UnitConverter_131/1  "<VINP_RADBHibeamIndication_flg>"
  UnitConverter_131/1 -> bus_creator/131  "VINP_RADBHibeamIndication_flg"
  bus_selector_1/114 -> UnitConverter_132/1  "<VINP_RADBOperationStatus_flg>"
  UnitConverter_132/1 -> bus_creator/132  "VINP_RADBOperationStatus_flg"
  bus_selector_1/115 -> UnitConverter_133/1  "<VINP_RADBWarning_flg>"
  UnitConverter_133/1 -> bus_creator/133  "VINP_RADBWarning_flg"
  bus_selector_1/116 -> UnitConverter_134/1  "<VINP_RAHBWarning_flg>"
  UnitConverter_134/1 -> bus_creator/134  "VINP_RAHBWarning_flg"
  bus_selector_1/117 -> UnitConverter_135/1  "<VINP_RDRLWarning_flg>"
  UnitConverter_135/1 -> bus_creator/135  "VINP_RDRLWarning_flg"
  bus_selector_1/118 -> UnitConverter_136/1  "<VINP_RLBWarning_flg>"
  UnitConverter_136/1 -> bus_creator/136  "VINP_RLBWarning_flg"
  bus_selector_1/119 -> UnitConverter_137/1  "<VINP_RpositionLampWarning_flg>"
  UnitConverter_137/1 -> bus_creator/137  "VINP_RpositionLampWarning_flg"
  bus_selector_1/120 -> UnitConverter_138/1  "<VINP_TrailerCheck_flg>"
  UnitConverter_138/1 -> bus_creator/138  "VINP_TrailerCheck_flg"
  bus_selector_1/121 -> UnitConverter_139/1  "<VINP_TrailerModeSta_enum>"
  UnitConverter_139/1 -> bus_creator/139  "VINP_TrailerModeSta_enum"
  bus_selector_1/122 -> UnitConverter_140/1  "<VINP_ZFRBCMChargerDoorSWSta_flg>"
  UnitConverter_140/1 -> bus_creator/140  "VINP_ZFRBCMChargerDoorSWSta_flg"
  bus_selector_1/123 -> UnitConverter_141/1  "<VINP_ZFRBCMHRLTurnLPNormalSta_flg>"
  UnitConverter_141/1 -> bus_creator/141  "VINP_ZFRBCMHRLTurnLPNormalSta_flg"
  bus_selector_1/124 -> UnitConverter_142/1  "<VINP_ZFRBCMHRRTurnLPHNormalSta_flg>"
  UnitConverter_142/1 -> bus_creator/142  "VINP_ZFRBCMHRRTurnLPHNormalSta_flg"
  bus_selector_1/125 -> UnitConverter_143/1  "<VINP_ZFRTHCMCLEVentActYSta_pct>"
  UnitConverter_143/1 -> bus_creator/143  "VINP_ZFRTHCMCLEVentActYSta_pct"
  bus_selector_1/126 -> UnitConverter_144/1  "<VINP_ZFRTHCMCREVentActYSta_pct>"
  UnitConverter_144/1 -> bus_creator/144  "VINP_ZFRTHCMCREVentActYSta_pct"
  bus_selector_1/127 -> UnitConverter_145/1  "<VINP_ZFRTHCMLEVentActYSta_pct>"
  UnitConverter_145/1 -> bus_creator/145  "VINP_ZFRTHCMLEVentActYSta_pct"
  bus_selector_1/128 -> UnitConverter_146/1  "<VINP_ZFRTHCMREVentActYSta_pct>"
  UnitConverter_146/1 -> bus_creator/146  "VINP_ZFRTHCMREVentActYSta_pct"
  bus_selector_1/129 -> UnitConverter_147/1  "<VINP_AGSErr_enum>"
  UnitConverter_147/1 -> bus_creator/147  "VINP_AGSErr_enum"
  bus_selector_1/130 -> UnitConverter_148/1  "<VINP_BatInTemp_C>"
  UnitConverter_148/1 -> bus_creator/148  "VINP_BatInTemp_C"
  bus_selector_1/131 -> UnitConverter_149/1  "<VINP_BatInTempErr_enum>"
  UnitConverter_149/1 -> bus_creator/149  "VINP_BatInTempErr_enum"
  bus_selector_1/132 -> UnitConverter_150/1  "<VINP_BatOutTemp_C>"
  UnitConverter_150/1 -> bus_creator/150  "VINP_BatOutTemp_C"
  bus_selector_1/133 -> UnitConverter_151/1  "<VINP_COMPErr_enum>"
  UnitConverter_151/1 -> bus_creator/151  "VINP_COMPErr_enum"
  bus_selector_1/134 -> UnitConverter_152/1  "<VINP_EACProtectEnable_enum>"
  UnitConverter_152/1 -> bus_creator/152  "VINP_EACProtectEnable_enum"
  bus_selector_1/135 -> UnitConverter_153/1  "<VINP_EWP3Err_enum>"
  UnitConverter_153/1 -> bus_creator/153  "VINP_EWP3Err_enum"
  bus_selector_1/136 -> UnitConverter_154/1  "<VINP_EXV1Err_enum>"
  UnitConverter_154/1 -> bus_creator/154  "VINP_EXV1Err_enum"
  bus_selector_1/137 -> UnitConverter_155/1  "<VINP_EXV2Err_enum>"
  UnitConverter_155/1 -> bus_creator/155  "VINP_EXV2Err_enum"
  bus_selector_1/138 -> UnitConverter_156/1  "<VINP_FanErr_enum>"
  UnitConverter_156/1 -> bus_creator/156  "VINP_FanErr_enum"
  bus_selector_1/139 -> UnitConverter_157/1  "<VINP_FrPMMLimpHomeActReq_flg>"
  UnitConverter_157/1 -> bus_creator/157  "VINP_FrPMMLimpHomeActReq_flg"
  bus_selector_1/140 -> UnitConverter_158/1  "<VINP_MotorInTemp_C>"
  UnitConverter_158/1 -> bus_creator/158  "VINP_MotorInTemp_C"
  bus_selector_1/141 -> UnitConverter_159/1  "<VINP_MotorInTempErr_enum>"
  UnitConverter_159/1 -> bus_creator/159  "VINP_MotorInTempErr_enum"
  bus_selector_1/142 -> UnitConverter_160/1  "<VINP_MotorOutTemp_C>"
  UnitConverter_160/1 -> bus_creator/160  "VINP_MotorOutTemp_C"
  bus_selector_1/143 -> UnitConverter_161/1  "<VINP_MotorOutTempErr_enum>"
  UnitConverter_161/1 -> bus_creator/161  "VINP_MotorOutTempErr_enum"
  bus_selector_1/144 -> UnitConverter_162/1  "<VINP_PTHighP_KPa>"
  UnitConverter_162/1 -> bus_creator/162  "VINP_PTHighP_KPa"
  bus_selector_1/145 -> UnitConverter_163/1  "<VINP_PTHighPErr_enum>"
  UnitConverter_163/1 -> bus_creator/163  "VINP_PTHighPErr_enum"
  bus_selector_1/146 -> UnitConverter_164/1  "<VINP_PTHighTact_C>"
  UnitConverter_164/1 -> bus_creator/164  "VINP_PTHighTact_C"
  bus_selector_1/147 -> UnitConverter_165/1  "<VINP_PTHighTactErr_enum>"
  UnitConverter_165/1 -> bus_creator/165  "VINP_PTHighTactErr_enum"
  bus_selector_1/148 -> UnitConverter_166/1  "<VINP_PTLowP1_KPa>"
  UnitConverter_166/1 -> bus_creator/166  "VINP_PTLowP1_KPa"
  bus_selector_1/149 -> UnitConverter_167/1  "<VINP_PTLowP1Err_enum>"
  UnitConverter_167/1 -> bus_creator/167  "VINP_PTLowP1Err_enum"
  bus_selector_1/150 -> UnitConverter_168/1  "<VINP_PTLowP2_KPa>"
  UnitConverter_168/1 -> bus_creator/168  "VINP_PTLowP2_KPa"
  bus_selector_1/151 -> UnitConverter_169/1  "<VINP_PTLowP2Err_enum>"
  UnitConverter_169/1 -> bus_creator/169  "VINP_PTLowP2Err_enum"
  bus_selector_1/152 -> UnitConverter_170/1  "<VINP_PTLowT1_C>"
  UnitConverter_170/1 -> bus_creator/170  "VINP_PTLowT1_C"
  bus_selector_1/153 -> UnitConverter_171/1  "<VINP_PTLowT1Err_enum>"
  UnitConverter_171/1 -> bus_creator/171  "VINP_PTLowT1Err_enum"
  bus_selector_1/154 -> UnitConverter_172/1  "<VINP_PTLowT2_C>"
  UnitConverter_172/1 -> bus_creator/172  "VINP_PTLowT2_C"
  bus_selector_1/155 -> UnitConverter_173/1  "<VINP_PTLowT2Err_enum>"
  UnitConverter_173/1 -> bus_creator/173  "VINP_PTLowT2Err_enum"
  bus_selector_1/156 -> UnitConverter_174/1  "<VINP_SOTXVErr_enum>"
  UnitConverter_174/1 -> bus_creator/174  "VINP_SOTXVErr_enum"
  bus_selector_1/157 -> UnitConverter_175/1  "<VINP_SOV1Err_enum>"
  UnitConverter_175/1 -> bus_creator/175  "VINP_SOV1Err_enum"
  bus_selector_1/158 -> UnitConverter_176/1  "<VINP_SOV2Err_enum>"
  UnitConverter_176/1 -> bus_creator/176  "VINP_SOV2Err_enum"
  bus_selector_1/159 -> UnitConverter_177/1  "<VINP_SOV3Err_enum>"
  UnitConverter_177/1 -> bus_creator/177  "VINP_SOV3Err_enum"
  bus_selector_1/160 -> UnitConverter_178/1  "<VINP_Tamb_C>"
  UnitConverter_178/1 -> bus_creator/178  "VINP_Tamb_C"
  bus_selector_1/161 -> UnitConverter_179/1  "<VINP_TambErr_enum>"
  UnitConverter_179/1 -> bus_creator/179  "VINP_TambErr_enum"
  bus_selector_1/162 -> UnitConverter_180/1  "<VINP_FrntPTCLeActHeatPwr_W>"
  UnitConverter_180/1 -> bus_creator/180  "VINP_FrntPTCLeActHeatPwr_W"
  bus_selector_1/163 -> UnitConverter_181/1  "<VINP_FrntPTCRearLeActHeatPwr_W>"
  UnitConverter_181/1 -> bus_creator/181  "VINP_FrntPTCRearLeActHeatPwr_W"
  bus_selector_1/164 -> UnitConverter_182/1  "<VINP_FrntPTCRearRiActHeatPwr_W>"
  UnitConverter_182/1 -> bus_creator/182  "VINP_FrntPTCRearRiActHeatPwr_W"
  bus_selector_1/165 -> UnitConverter_183/1  "<VINP_FrntPTCRiActHeatPwr_W>"
  UnitConverter_183/1 -> bus_creator/183  "VINP_FrntPTCRiActHeatPwr_W"
  bus_selector_1/166 -> UnitConverter_184/1  "<VINP_COMPActualPwr_W>"
  UnitConverter_184/1 -> bus_creator/184  "VINP_COMPActualPwr_W"
  bus_selector_1/167 -> UnitConverter_185/1  "<VINP_COMPConCur_A>"
  UnitConverter_185/1 -> bus_creator/185  "VINP_COMPConCur_A"
  bus_selector_1/168 -> UnitConverter_186/1  "<VINP_COMPConVolt_V>"
  UnitConverter_186/1 -> bus_creator/186  "VINP_COMPConVolt_V"
  bus_selector_1/169 -> UnitConverter_187/1  "<VINP_COMPStatorSpd_rpm>"
  UnitConverter_187/1 -> bus_creator/187  "VINP_COMPStatorSpd_rpm"
  bus_selector_1/170 -> UnitConverter_188/1  "<VINP_PTC1PowerConsumption_kW>"
  UnitConverter_188/1 -> bus_creator/188  "VINP_PTC1PowerConsumption_kW"
  bus_selector_1/171 -> UnitConverter_189/1  "<VINP_CSWDimSw_flg>"
  UnitConverter_189/1 -> bus_creator/189  "VINP_CSWDimSw_flg"
  bus_selector_1/172 -> UnitConverter_190/1  "<VINP_CSWFWasSwSta_enum>"
  UnitConverter_190/1 -> bus_creator/190  "VINP_CSWFWasSwSta_enum"
  bus_selector_1/173 -> UnitConverter_191/1  "<VINP_CSWFWipSwSta_enum>"
  UnitConverter_191/1 -> bus_creator/191  "VINP_CSWFWipSwSta_enum"
  bus_selector_1/174 -> UnitConverter_192/1  "<VINP_CSWPassSWSta_flg>"
  UnitConverter_192/1 -> bus_creator/192  "VINP_CSWPassSWSta_flg"
  bus_selector_1/175 -> UnitConverter_193/1  "<VINP_CSWRWasSWSta_enum>"
  UnitConverter_193/1 -> bus_creator/193  "VINP_CSWRWasSWSta_enum"
  bus_selector_1/176 -> UnitConverter_194/1  "<VINP_CSWRWipIntSwSta_enum>"
  UnitConverter_194/1 -> bus_creator/194  "VINP_CSWRWipIntSwSta_enum"
  bus_selector_1/177 -> UnitConverter_195/1  "<VINP_CSWTurnSwSta_enum>"
  UnitConverter_195/1 -> bus_creator/195  "VINP_CSWTurnSwSta_enum"
  bus_selector_1/178 -> UnitConverter_196/1  "<VINP_FAPWL01LINResponseError_flg>"
  UnitConverter_196/1 -> bus_creator/196  "VINP_FAPWL01LINResponseError_flg"
  bus_selector_1/179 -> UnitConverter_197/1  "<VINP_LDrvMotorRelayError_flg>"
  UnitConverter_197/1 -> bus_creator/197  "VINP_LDrvMotorRelayError_flg"
  bus_selector_1/180 -> UnitConverter_198/1  "<VINP_LDrvMotorRippleError_flg>"
  UnitConverter_198/1 -> bus_creator/198  "VINP_LDrvMotorRippleError_flg"
  bus_selector_1/181 -> UnitConverter_199/1  "<VINP_LDrvValWdwOpened_pct>"
  UnitConverter_199/1 -> bus_creator/199  "VINP_LDrvValWdwOpened_pct"
  bus_selector_1/182 -> UnitConverter_200/1  "<VINP_LDrvWdwPositionSts_enum>"
  UnitConverter_200/1 -> bus_creator/200  "VINP_LDrvWdwPositionSts_enum"
  bus_selector_1/183 -> UnitConverter_201/1  "<VINP_LPasMotorRelayError_flg>"
  UnitConverter_201/1 -> bus_creator/201  "VINP_LPasMotorRelayError_flg"
  bus_selector_1/184 -> UnitConverter_202/1  "<VINP_LPasMotorRippleError_flg>"
  UnitConverter_202/1 -> bus_creator/202  "VINP_LPasMotorRippleError_flg"
  bus_selector_1/185 -> UnitConverter_203/1  "<VINP_LPasValWdwOpened_pct>"
  UnitConverter_203/1 -> bus_creator/203  "VINP_LPasValWdwOpened_pct"
  bus_selector_1/186 -> UnitConverter_204/1  "<VINP_LPasWdwPositionSts_enum>"
  UnitConverter_204/1 -> bus_creator/204  "VINP_LPasWdwPositionSts_enum"
  bus_selector_1/187 -> UnitConverter_205/1  "<VINP_LRLDMotorRelayError_flg>"
  UnitConverter_205/1 -> bus_creator/205  "VINP_LRLDMotorRelayError_flg"
  bus_selector_1/188 -> UnitConverter_206/1  "<VINP_LRLDMotorRippleError_flg>"
  UnitConverter_206/1 -> bus_creator/206  "VINP_LRLDMotorRippleError_flg"
  bus_selector_1/189 -> UnitConverter_207/1  "<VINP_LRLDValWdwOpened_pct>"
  UnitConverter_207/1 -> bus_creator/207  "VINP_LRLDValWdwOpened_pct"
  bus_selector_1/190 -> UnitConverter_208/1  "<VINP_LRLDWdwPositionSts_enum>"
  UnitConverter_208/1 -> bus_creator/208  "VINP_LRLDWdwPositionSts_enum"
  bus_selector_1/191 -> UnitConverter_209/1  "<VINP_LRRDMotorRelayError_flg>"
  UnitConverter_209/1 -> bus_creator/209  "VINP_LRRDMotorRelayError_flg"
  bus_selector_1/192 -> UnitConverter_210/1  "<VINP_LRRDMotorRippleError_flg>"
  UnitConverter_210/1 -> bus_creator/210  "VINP_LRRDMotorRippleError_flg"
  bus_selector_1/193 -> UnitConverter_211/1  "<VINP_LRRDValWdwOpened_pct>"
  UnitConverter_211/1 -> bus_creator/211  "VINP_LRRDValWdwOpened_pct"
  bus_selector_1/194 -> UnitConverter_212/1  "<VINP_LRRDWdwPositionSts_enum>"
  UnitConverter_212/1 -> bus_creator/212  "VINP_LRRDWdwPositionSts_enum"
  bus_selector_1/195 -> UnitConverter_213/1  "<VINP_RAPWL01LINResponseError_flg>"
  UnitConverter_213/1 -> bus_creator/213  "VINP_RAPWL01LINResponseError_flg"
  bus_selector_1/196 -> UnitConverter_214/1  "<VINP_RLSLampSta_flg>"
  UnitConverter_214/1 -> bus_creator/214  "VINP_RLSLampSta_flg"
  bus_selector_1/197 -> UnitConverter_215/1  "<VINP_RLSRainSnrWiperCmd_enum>"
  UnitConverter_215/1 -> bus_creator/215  "VINP_RLSRainSnrWiperCmd_enum"
  bus_selector_1/198 -> UnitConverter_216/1  "<VINP_SWC2LADASSta_flg>"
  UnitConverter_216/1 -> bus_creator/216  "VINP_SWC2LADASSta_flg"
  bus_selector_1/199 -> UnitConverter_217/1  "<VINP_SWC2LDriveModeSta_flg>"
  UnitConverter_217/1 -> bus_creator/217  "VINP_SWC2LDriveModeSta_flg"
  bus_selector_1/200 -> UnitConverter_218/1  "<VINP_SWC2LHomeSta_flg>"
  UnitConverter_218/1 -> bus_creator/218  "VINP_SWC2LHomeSta_flg"
  bus_selector_1/201 -> UnitConverter_219/1  "<VINP_SWC2LLeftSta_flg>"
  UnitConverter_219/1 -> bus_creator/219  "VINP_SWC2LLeftSta_flg"
  bus_selector_1/202 -> UnitConverter_220/1  "<VINP_SWC2LRegenUpSta_flg>"
  UnitConverter_220/1 -> bus_creator/220  "VINP_SWC2LRegenUpSta_flg"
  bus_selector_1/203 -> UnitConverter_221/1  "<VINP_SWC2LRightSta_flg>"
  UnitConverter_221/1 -> bus_creator/221  "VINP_SWC2LRightSta_flg"
  bus_selector_1/204 -> UnitConverter_222/1  "<VINP_SWC2LScrollDownSta_flg>"
  UnitConverter_222/1 -> bus_creator/222  "VINP_SWC2LScrollDownSta_flg"
  bus_selector_1/205 -> UnitConverter_223/1  "<VINP_SWC2LScrollPressSta_flg>"
  UnitConverter_223/1 -> bus_creator/223  "VINP_SWC2LScrollPressSta_flg"
  bus_selector_1/206 -> UnitConverter_224/1  "<VINP_SWC2LScrollUpSta_flg>"
  UnitConverter_224/1 -> bus_creator/224  "VINP_SWC2LScrollUpSta_flg"
  bus_selector_1/207 -> UnitConverter_225/1  "<VINP_SWC2RCustomizeSta_flg>"
  UnitConverter_225/1 -> bus_creator/225  "VINP_SWC2RCustomizeSta_flg"
  bus_selector_1/208 -> UnitConverter_226/1  "<VINP_SWC2RLeftSta_flg>"
  UnitConverter_226/1 -> bus_creator/226  "VINP_SWC2RLeftSta_flg"
  bus_selector_1/209 -> UnitConverter_227/1  "<VINP_SWC2RPageSwitchSta_flg>"
  UnitConverter_227/1 -> bus_creator/227  "VINP_SWC2RPageSwitchSta_flg"
  bus_selector_1/210 -> UnitConverter_228/1  "<VINP_SWC2RRegenDownSta_flg>"
  UnitConverter_228/1 -> bus_creator/228  "VINP_SWC2RRegenDownSta_flg"
  bus_selector_1/211 -> UnitConverter_229/1  "<VINP_SWC2RRightSta_flg>"
  UnitConverter_229/1 -> bus_creator/229  "VINP_SWC2RRightSta_flg"
  bus_selector_1/212 -> UnitConverter_230/1  "<VINP_SWC2RScrollDownSta_flg>"
  UnitConverter_230/1 -> bus_creator/230  "VINP_SWC2RScrollDownSta_flg"
  bus_selector_1/213 -> UnitConverter_231/1  "<VINP_SWC2RScrollPressSta_flg>"
  UnitConverter_231/1 -> bus_creator/231  "VINP_SWC2RScrollPressSta_flg"
  bus_selector_1/214 -> UnitConverter_232/1  "<VINP_SWC2RScrollUpSta_flg>"
  UnitConverter_232/1 -> bus_creator/232  "VINP_SWC2RScrollUpSta_flg"
  bus_selector_1/215 -> UnitConverter_233/1  "<VINP_SWC2RVRSta_flg>"
  UnitConverter_233/1 -> bus_creator/233  "VINP_SWC2RVRSta_flg"
  bus_selector_1/216 -> UnitConverter_234/1  "<VINP_SWCACCSta_flg>"
  UnitConverter_234/1 -> bus_creator/234  "VINP_SWCACCSta_flg"
  bus_selector_1/217 -> UnitConverter_235/1  "<VINP_SWCCANCELSta_flg>"
  UnitConverter_235/1 -> bus_creator/235  "VINP_SWCCANCELSta_flg"
  bus_selector_1/218 -> UnitConverter_236/1  "<VINP_SWCDistanceSta_flg>"
  UnitConverter_236/1 -> bus_creator/236  "VINP_SWCDistanceSta_flg"
  bus_selector_1/219 -> UnitConverter_237/1  "<VINP_SWCDownSta_flg>"
  UnitConverter_237/1 -> bus_creator/237  "VINP_SWCDownSta_flg"
  bus_selector_1/220 -> UnitConverter_238/1  "<VINP_SWCLKASta_flg>"
  UnitConverter_238/1 -> bus_creator/238  "VINP_SWCLKASta_flg"
  bus_selector_1/221 -> UnitConverter_239/1  "<VINP_SWCLeftSta_flg>"
  UnitConverter_239/1 -> bus_creator/239  "VINP_SWCLeftSta_flg"
  bus_selector_1/222 -> UnitConverter_240/1  "<VINP_SWCRegenDown_flg>"
  UnitConverter_240/1 -> bus_creator/240  "VINP_SWCRegenDown_flg"
  bus_selector_1/223 -> UnitConverter_241/1  "<VINP_SWCRegenUp_flg>"
  UnitConverter_241/1 -> bus_creator/241  "VINP_SWCRegenUp_flg"
  bus_selector_1/224 -> UnitConverter_242/1  "<VINP_SWCResUpSta_flg>"
  UnitConverter_242/1 -> bus_creator/242  "VINP_SWCResUpSta_flg"
  bus_selector_1/225 -> UnitConverter_243/1  "<VINP_SWCRightSta_flg>"
  UnitConverter_243/1 -> bus_creator/243  "VINP_SWCRightSta_flg"
  bus_selector_1/226 -> UnitConverter_244/1  "<VINP_SWCSetdownSta_flg>"
  UnitConverter_244/1 -> bus_creator/244  "VINP_SWCSetdownSta_flg"
  bus_selector_1/227 -> UnitConverter_245/1  "<VINP_SWCTripSta_flg>"
  UnitConverter_245/1 -> bus_creator/245  "VINP_SWCTripSta_flg"
  bus_selector_1/228 -> UnitConverter_246/1  "<VINP_SWCUndefinedSta_flg>"
  UnitConverter_246/1 -> bus_creator/246  "VINP_SWCUndefinedSta_flg"
  bus_selector_1/229 -> UnitConverter_247/1  "<VINP_SWCUpSta_flg>"
  UnitConverter_247/1 -> bus_creator/247  "VINP_SWCUpSta_flg"
  bus_selector_1/230 -> UnitConverter_248/1  "<VINP_SWCVRSta_flg>"
  UnitConverter_248/1 -> bus_creator/248  "VINP_SWCVRSta_flg"
  bus_selector_1/231 -> UnitConverter_249/1  "<VINP_SWCmodeSta_flg>"
  UnitConverter_249/1 -> bus_creator/249  "VINP_SWCmodeSta_flg"
  bus_selector_1/232 -> UnitConverter_250/1  "<VINP_ACT1ResponseError_flg>"
  UnitConverter_250/1 -> bus_creator/250  "VINP_ACT1ResponseError_flg"
  bus_selector_1/233 -> UnitConverter_251/1  "<VINP_AGSActualPosition_enum>"
  UnitConverter_251/1 -> bus_creator/251  "VINP_AGSActualPosition_enum"
  bus_selector_1/234 -> UnitConverter_252/1  "<VINP_FGSIntenRspSta_enum>"
  UnitConverter_252/1 -> bus_creator/252  "VINP_FGSIntenRspSta_enum"
  bus_selector_1/235 -> UnitConverter_253/1  "<VINP_EWP1BlockError_enum>"
  UnitConverter_253/1 -> bus_creator/253  "VINP_EWP1BlockError_enum"
  bus_selector_1/236 -> UnitConverter_254/1  "<VINP_EWP1OverCurrError_enum>"
  UnitConverter_254/1 -> bus_creator/254  "VINP_EWP1OverCurrError_enum"
  bus_selector_1/237 -> UnitConverter_255/1  "<VINP_EWP2BlockError_enum>"
  UnitConverter_255/1 -> bus_creator/255  "VINP_EWP2BlockError_enum"
  bus_selector_1/238 -> UnitConverter_256/1  "<VINP_EWP2OverCurrError_enum>"
  UnitConverter_256/1 -> bus_creator/256  "VINP_EWP2OverCurrError_enum"
  bus_selector_1/239 -> UnitConverter_257/1  "<VINP_EWP3BlockError_enum>"
  UnitConverter_257/1 -> bus_creator/257  "VINP_EWP3BlockError_enum"
  bus_selector_1/240 -> UnitConverter_258/1  "<VINP_EWP3OverCurrError_enum>"
  UnitConverter_258/1 -> bus_creator/258  "VINP_EWP3OverCurrError_enum"
  bus_selector_1/241 -> UnitConverter_259/1  "<VINP_DSEATAntiSta_flg>"
  UnitConverter_259/1 -> bus_creator/259  "VINP_DSEATAntiSta_flg"
  bus_selector_1/242 -> UnitConverter_260/1  "<VINP_DSEATEntryFunSta_flg>"
  UnitConverter_260/1 -> bus_creator/260  "VINP_DSEATEntryFunSta_flg"
  bus_selector_1/243 -> UnitConverter_261/1  "<VINP_DSEATErrorSta_flg>"
  UnitConverter_261/1 -> bus_creator/261  "VINP_DSEATErrorSta_flg"
  bus_selector_1/244 -> UnitConverter_262/1  "<VINP_DSEATHWVer_enum>"
  UnitConverter_262/1 -> bus_creator/262  "VINP_DSEATHWVer_enum"
  bus_selector_1/245 -> UnitConverter_263/1  "<VINP_DSEATMode_enum>"
  UnitConverter_263/1 -> bus_creator/263  "VINP_DSEATMode_enum"
  bus_selector_1/246 -> UnitConverter_264/1  "<VINP_DSEATSWVer_enum>"
  UnitConverter_264/1 -> bus_creator/264  "VINP_DSEATSWVer_enum"
  bus_selector_1/247 -> UnitConverter_265/1  "<VINP_DSEATVentSta_enum>"
  UnitConverter_265/1 -> bus_creator/265  "VINP_DSEATVentSta_enum"
  bus_selector_1/248 -> UnitConverter_266/1  "<VINP_DSEATheatersta_enum>"
  UnitConverter_266/1 -> bus_creator/266  "VINP_DSEATheatersta_enum"
  bus_selector_1/249 -> UnitConverter_267/1  "<VINP_PSEATErrorSta_flg>"
  UnitConverter_267/1 -> bus_creator/267  "VINP_PSEATErrorSta_flg"
  bus_selector_1/250 -> UnitConverter_268/1  "<VINP_PSEATHWVer_enum>"
  UnitConverter_268/1 -> bus_creator/268  "VINP_PSEATHWVer_enum"
  bus_selector_1/251 -> UnitConverter_269/1  "<VINP_PSEATMode_enum>"
  UnitConverter_269/1 -> bus_creator/269  "VINP_PSEATMode_enum"
  bus_selector_1/252 -> UnitConverter_270/1  "<VINP_PSEATSWVer_enum>"
  UnitConverter_270/1 -> bus_creator/270  "VINP_PSEATSWVer_enum"
  bus_selector_1/253 -> UnitConverter_271/1  "<VINP_PSEATVentSta_enum>"
  UnitConverter_271/1 -> bus_creator/271  "VINP_PSEATVentSta_enum"
  bus_selector_1/254 -> UnitConverter_272/1  "<VINP_PSEATheatersta_enum>"
  UnitConverter_272/1 -> bus_creator/272  "VINP_PSEATheatersta_enum"
  [inp_CanValid_bus] -> bus_selector/1
  [inp_Hal_bus] -> bus_selector_1/1
  bus_creator/1 -> BINP_outputs/1
